simulink model "velo_pi"  (Simulink 8.7)
settings: Solver=FixedStepAuto  StartTime=0.0  StopTime=10.0  RelTol=1e-3
undefined symbols (not defined in the file): ts
libraries: arduinolib x3
settings Model: Creator=morita  LastModifiedBy=morita  SimulationMode=external  ExtModeTrigDuration=2
settings DataIOCC: LimitDataPoints=off  SaveFormat=Dataset
settings OptimizationCC: OptimizeModelRefInitCode=on  LifeSpan=1  MaxStackSize=64
settings DebuggingCC: UnderspecifiedInitializationDetection=Simplified  MergeDetectMultiDrivingBlocksExec=error
settings HardwareCC: ProdBitPerInt=16  ProdBitPerPointer=16  ProdIntDivRoundTo=Zero  ProdEndianess=LittleEndian  ProdWordSize=8  ProdHWDeviceType=Atmel->AVR  UseEmbeddedCoderFeatures=off  UseSimulinkCoderFeatures=off
settings ModelReferenceCC: PropagateSignalLabelsOutOfModel=on
settings RTWCC: SystemTargetFile=ert.tlc  HardwareBoard=Arduino Mega 2560  TLCOptions=-aInlineSetEventsForThisBaseRateFcn=TLC_FALSE -aSuppressMultiTaskScheduler=TLC_FALSE  TemplateMakefile=ert_default_tmf  Description=Embedded Coder  GenerateReport=on  Toolchain=Arduino AVR v1.6.1  BuildConfiguration=Faster Runs  IncludeHyperlinkInReport=on  LaunchReport=on  GenerateTraceInfo=on  GenerateTraceReport=on  GenerateTraceReportSl=on  GenerateTraceReportSf=on  GenerateTraceReportEml=on
settings MATStruct: className=codertarget.tools.BuildHook  argsTopModelOnly=[]  excludedModels=[]  includeReferencedModels=on  includeTopModel=on  enabled=on  UseCoderTarget=[1]  TargetHardware=Arduino Mega 2560  RTOS=Baremetal  Scheduler_interrupt_source=[0.0]  DataVersion=2016.02  Baudrate=115200  COMPort=codertarget.arduinobase.internal.getExternalModeMexArgs('Serial')  Verbose=[0]  IPAddress=codertarget.arduinobase.internal.getExternalModeMexArgs('Ethernet')  Port=17725  Configuration=Serial  BuildAction=Build, load and run  Set_host_COM_port=Automatically  COM_port_number=1  Enable_overrun_detection=[0.0]  Digital_output_to_set_on_overrun=13  Analog_input_reference_voltage=[0.0]  Serial0_baud_rate=9600  Serial1_baud_rate=9600  Serial2_baud_rate=9600  Serial3_baud_rate=9600  SPI_clock_out_frequency=4000  SPI_mode=Mode 0 - Clock Polarity 0, Clock Phase 0  SPI_bitorder=MSB first  Disable_DHCP_Ethernet=[0.0]  Local_ip_address=192.168.0.20  Local_mac_address=DE:AD:BE:EF:FE:ED  Disable_DHCP_Wifi=[0.0]  Wifi_ip_address=192.168.1.20  Wifi_SSID=yourNetwork  Set_Wifi_Encryption=None  Wifi_WEP_key=D0D0DEADF00DABBADEAFBEADED  Wifi_WEP_key_index=0  Wifi_WPA_password=secretPassword
settings CodeAppCC: ForceParamTrailComments=on  IgnoreCustomStorageClasses=off  OperatorAnnotations=on  SimulinkDataObjDesc=on  SFDataObjDesc=on  MATLABFcnDesc=on  InsertBlockDesc=on  MATLABSourceComments=on
settings ERTTargetCC: MultiwordLength=2048  SupportContinuousTime=on  SupportNonInlinedSFcns=on  SupportVariableSizeSignals=on
settings ConfigComp: CovModelRefEnable=off

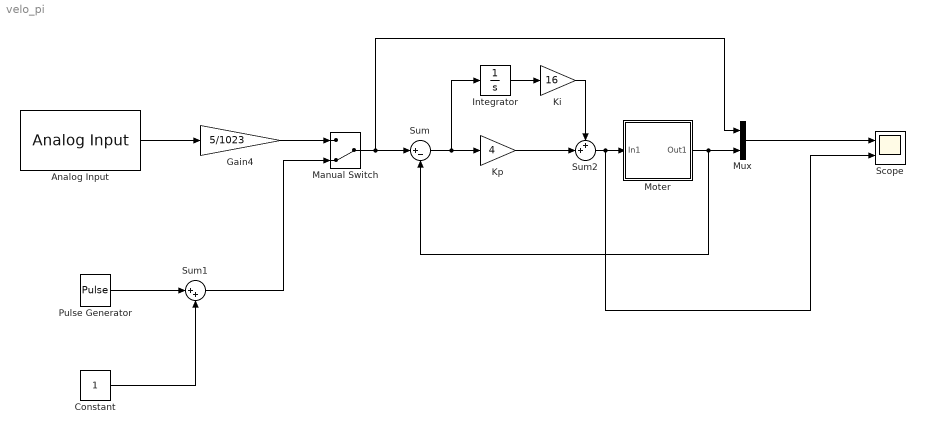
== system velo_pi ==
  Analog Input : arduinolib/Analog Input  pinNumber=1  sampleTime=ts  blockPlatform=arduino
  Constant : Constant
  Gain4 : Gain  Gain=5/1023
  Integrator : Integrator
  Ki : Gain  Gain=16  ParamDataTypeStr=double
  Kp : Gain  Gain=4  ParamDataTypeStr=double
  Manual Switch : ManualSwitch  CurrentSetting=0
  Moter : Subsystem
  Mux : Mux  Inputs=2
  Pulse Generator : DiscretePulseGenerator  Amplitude=0.5  Period=10/ts  PulseWidth=5/ts  SampleTime=ts
  Scope : Scope  NumInputPorts=2
  Sum : Sum  Inputs=|+-
  Sum1 : Sum  Inputs=|++
  Sum2 : Sum  Inputs=++|
  wires:
  Analog Input/1 -> Gain4/1
  Mux/1 -> Scope/1
  Gain4/1 -> Manual Switch/1
  Sum/1 -> Kp/1, Integrator/1
  Manual Switch/1 -> Mux/1, Sum/1
  Moter/1(Out1) -> Mux/2, Sum/2
  Pulse Generator/1 -> Sum1/1
  Constant/1 -> Sum1/2
  Sum1/1 -> Manual Switch/2
  Integrator/1 -> Ki/1
  Sum2/1 -> Scope/2, Moter/1(In1)
  Ki/1 -> Sum2/1
  Kp/1 -> Sum2/2

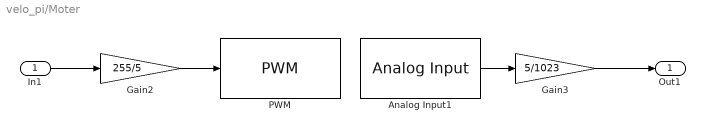
== system velo_pi/Moter ==
  In1 : Inport
  Analog Input1 : arduinolib/Analog Input  pinNumber=0  sampleTime=ts  blockPlatform=arduino
  Gain2 : Gain  Gain=255/5  ParamDataTypeStr=double  OutDataTypeStr=double
  Gain3 : Gain  Gain=5/1023  ParamDataTypeStr=double  OutDataTypeStr=double
  PWM : arduinolib/PWM  pinNumber=3  blockPlatform=arduino
  Out1 : Outport  OutDataTypeStr=double
  wires:
  Analog Input1/1 -> Gain3/1
  Gain3/1 -> Out1/1
  Gain2/1 -> PWM/1
  In1/1 -> Gain2/1
